simulink model "Simulink_P3"  (R2025a)
settings: Solver=VariableStepAuto  StartTime=0.0  StopTime=10.0  RelTol=1e-3
InitFcn:
  | m1 = 290
  | b1 = 1000
  | m2 = 59
  | k1 = 16182
  | f = 0
  | k2 = 19000

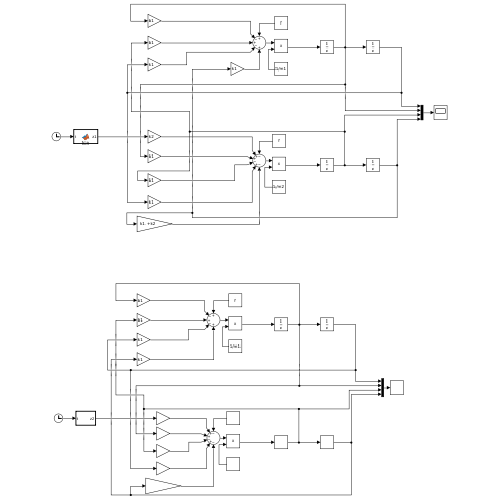
[thumbnail: Simulink's stored preview of the top-level diagram]
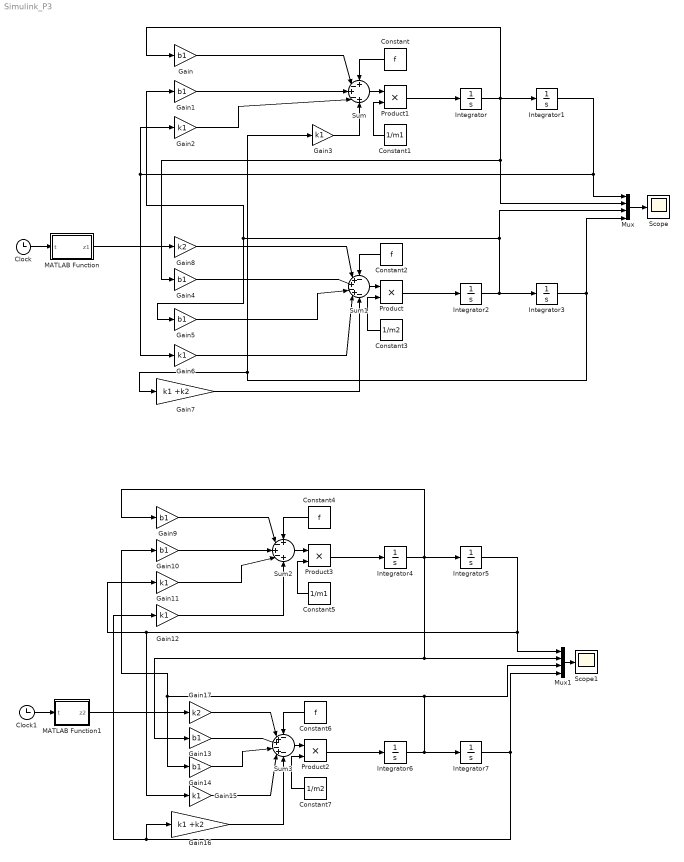
== system Simulink_P3 ==
  Clock : Clock
  Clock1 : Clock
  Constant{,2,4,6} (4 alike) : Constant  Value=f
  Constant1 : Constant  Value=1/m1
  Constant3 : Constant  Value=1/m2
  Constant5 : Constant  Value=1/m1
  Constant7 : Constant  Value=1/m2
  Gain{,1,4..5,9..10,13..14} (8 alike) : Gain  Gain=b1
  Gain{2..3,6,11..12,15} (6 alike) : Gain  Gain=k1
  Gain16 : Gain  Gain=k1 +k2
  Gain17 : Gain  Gain=k2
  Gain7 : Gain  Gain=k1 +k2
  Gain8 : Gain  Gain=k2
  Integrator{,1..7} (8 alike) : Integrator
  MATLAB Function : MATLAB Function  TreatAsAtomicUnit=on
  MATLAB Function1 : MATLAB Function  TreatAsAtomicUnit=on
  Mux : Mux
  Mux1 : Mux
  Product{,1..3} (4 alike) : Product
  Scope : Scope
      settings: ActiveDisplayYMinimum=-0.14349624487296697  ActiveDisplayYMaximum=0.16132544391466044
  Scope1 : Scope
      settings: ActiveDisplayYMinimum=-0.56212847550380984  ActiveDisplayYMaximum=0.3473951795246904
  Sum : Sum  Inputs=+-+-+
  Sum1 : Sum  Inputs=-++-+-
  Sum2 : Sum  Inputs=+-+-+
  Sum3 : Sum  Inputs=-++-+-
  wires:
  Integrator3/1 -> Gain3/1, Gain7/1, Mux/4
  Integrator4/1 -> Integrator5/1, Gain9/1, Gain13/1, Mux1/2
  Constant2/1 -> Sum1/1
  Gain6/1 -> Sum1/5
  Gain3/1 -> Sum/5
  Clock1/1 -> MATLAB Function1/1(t)
  Sum1/1 -> Product/1
  Product/1 -> Integrator2/1
  Gain/1 -> Sum/2
  Integrator1/1 -> Gain6/1, Gain2/1, Mux/1
  Integrator7/1 -> Gain12/1, Gain16/1, Mux1/4
  Constant3/1 -> Product/2
  Integrator/1 -> Integrator1/1, Gain/1, Gain4/1, Mux/2
  Mux/1 -> Scope/1
  Gain15/1 -> Sum3/5
  Gain10/1 -> Sum2/3
  Gain13/1 -> Sum3/3
  Gain7/1 -> Sum1/6
  Constant4/1 -> Sum2/1
  Integrator6/1 -> Gain14/1, Gain10/1, Mux1/3, Integrator7/1
  Integrator2/1 -> Gain5/1, Gain1/1, Mux/3, Integrator3/1
  Clock/1 -> MATLAB Function/1(t)
  Gain12/1 -> Sum2/5
  Integrator5/1 -> Gain15/1, Gain11/1, Mux1/1
  Product1/1 -> Integrator/1
  Product2/1 -> Integrator6/1
  Gain11/1 -> Sum2/4
  Gain16/1 -> Sum3/6
  MATLAB Function1/1(z2) -> Gain17/1
  Constant6/1 -> Sum3/1
  Gain8/1 -> Sum1/2
  Constant1/1 -> Product1/2
  Constant/1 -> Sum/1
  Sum/1 -> Product1/1
  Gain9/1 -> Sum2/2
  Sum2/1 -> Product3/1
  Gain2/1 -> Sum/4
  Gain5/1 -> Sum1/4
  Constant5/1 -> Product3/2
  Product3/1 -> Integrator4/1
  Sum3/1 -> Product2/1
  Constant7/1 -> Product2/2
  Gain17/1 -> Sum3/2
  Gain1/1 -> Sum/3
  Mux1/1 -> Scope1/1
  MATLAB Function/1(z1) -> Gain8/1
  Gain4/1 -> Sum1/3
  Gain14/1 -> Sum3/4

== matlab function Simulink_P3/MATLAB Function ==
  data: t input; z1 output
function z1 = fcn(t)
z1 = 0.05*sin(0.5*pi*t)

== matlab function Simulink_P3/MATLAB Function1 ==
  data: t input; z2 output
function z2 = fcn(t)
z2 = 0.05*sin(20*pi*t)
